simulink model "simpleMassSipringDamperModel_steadySpace"  (R2020b)
settings: Solver=FixedStepAuto  StartTime=0.0  StopTime=10.0  FixedStep=1e-3  RelTol=1e-3
settings Model: Creator=kuzub  LastModifiedBy=kuzub

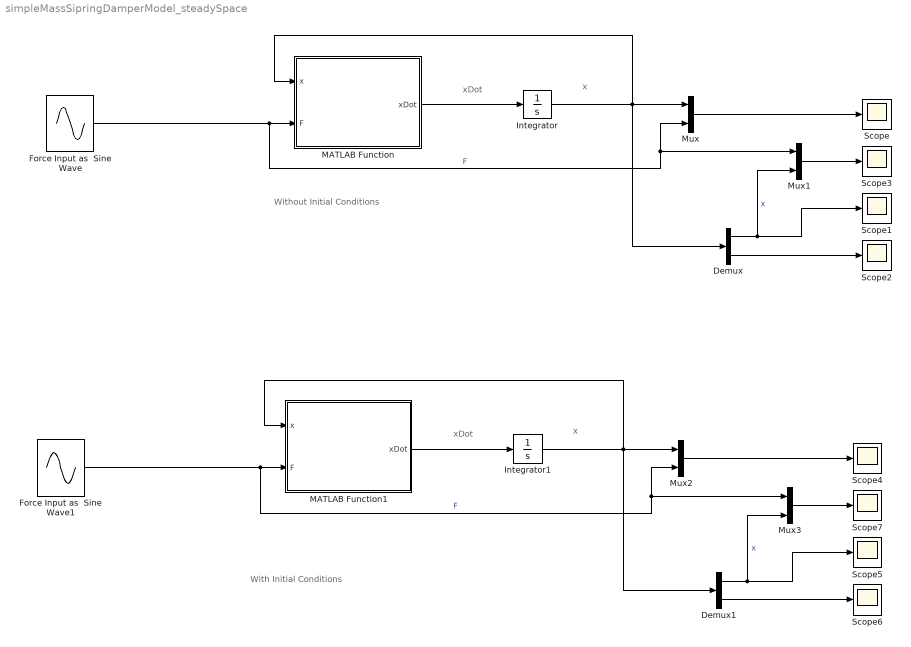
== system simpleMassSipringDamperModel_steadySpace ==
  note: With Initial Conditions
  note: x
  note: xDot
  note: x
  note: xDot
  note: Without Initial Conditions
  Demux : Demux  Outputs=2
  Demux1 : Demux  Outputs=2
  Force Input as  Sine Wave : Sin  Amplitude=5  Bias=5  Frequency=2*pi*1  SampleTime=0
  Force Input as  Sine Wave1 : Sin  Amplitude=5  Bias=5  Frequency=2*pi*1  SampleTime=0
  Integrator : Integrator  InitialCondition=[0;0]
  Integrator1 : Integrator  InitialCondition=[0;0]
  MATLAB Function : MATLAB Function  TreatAsAtomicUnit=on
  MATLAB Function1 : MATLAB Function  TreatAsAtomicUnit=on
  Mux{,1..3} (4 alike) : Mux  Inputs=2
  Scope{,1..7} (8 alike) : Scope
  wires:
  MATLAB Function/1(xDot) -> Integrator/1
  Integrator/1 -> Demux/1, MATLAB Function/1(x), Mux/1
  Mux/1 -> Scope/1
  Force Input as  Sine Wave/1 -> Mux1/1, Mux/2, MATLAB Function/2(F)  "F"
  Demux/1 -> Mux1/2, Scope1/1  "x"
  Demux/2 -> Scope2/1
  Mux1/1 -> Scope3/1
  Mux3/1 -> Scope7/1
  Demux1/2 -> Scope6/1
  Demux1/1 -> Scope5/1, Mux3/2  "x"
  Force Input as  Sine Wave1/1 -> MATLAB Function1/2(F), Mux2/2, Mux3/1  "F"
  Mux2/1 -> Scope4/1
  Integrator1/1 -> Mux2/1, MATLAB Function1/1(x), Demux1/1
  MATLAB Function1/1(xDot) -> Integrator1/1

== matlab function simpleMassSipringDamperModel_steadySpace/MATLAB Function ==
  data: x input; xDot output; F input
function xDot = fcn(x, F)

%   Constant Variables
    m = 2;  %kg
    c = 2;  %N/ms
    k = 2;  %N/m

    A = [0,  1;
         -k/m,  -c/m];
     
    B = [0;
         1/m];
     
     
    xDot = A*x + B*F;


end

== matlab function simpleMassSipringDamperModel_steadySpace/MATLAB Function1 ==
  data: x input; xDot output; F input
function xDot = fcn(x, F)

%   Constant Variables
    m = 2;  %kg
    c = 2;  %N/ms
    k = 2;  %N/m

    A = [0,  1;
         -k/m,  -c/m];
     
    B = [0;
         1/m];
     
     
    xDot = A*x + B*F;


end
